simulink model "simulator_v1"  (R2025b)
settings: Solver=VariableStepAuto  StartTime=0.0  StopTime=10.0  RelTol=1e-3
values from neighbouring files (symbols this model uses):
  att_ctrl = struct    [parametrosCarga4x.m]
  payload = struct    [parametrosCarga4x.m]
  pos_ctrl = struct    [parametrosCarga4x.m]
libraries: ASK x2
settings Model: Creator=ateveraz  LastModifiedBy=ateveraz

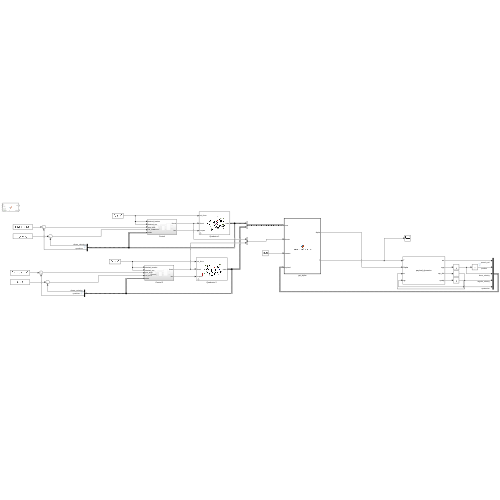
[thumbnail: Simulink's stored preview of the top-level diagram]
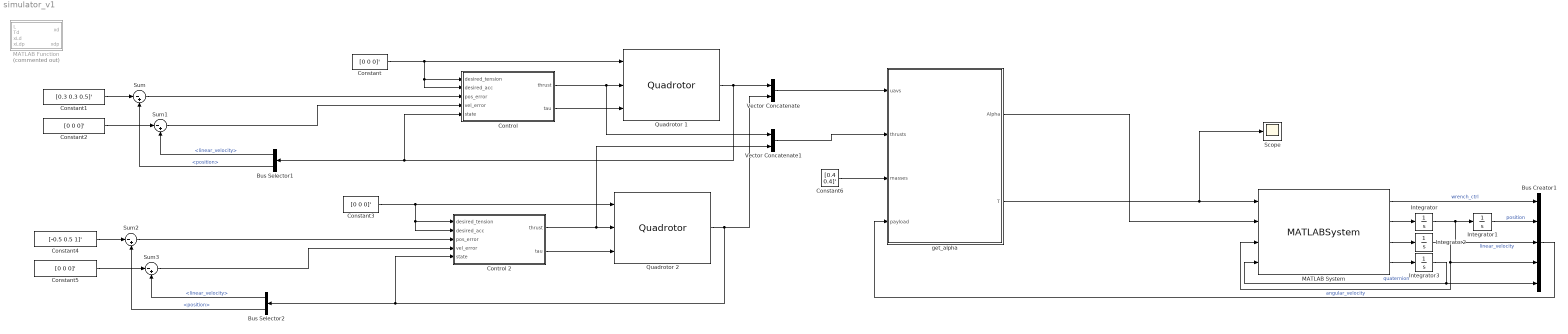
== system simulator_v1 ==
  Bus Creator1 : BusCreator  Inputs=5  OutDataTypeStr=Bus: payload_state  NonVirtualBus=on
  Bus Selector1 : BusSelector  OutputSignals=linear_velocity,position
  Bus Selector2 : BusSelector  OutputSignals=linear_velocity,position
  Constant{,2..3,5} (4 alike) : Constant  Value=[0 0 0]'
  Constant1 : Constant  Value=[0.3 0.3 0.5]'
  Constant4 : Constant  Value=[-0.5 0.5 1]'
  Constant6 : Constant  Value=[0.4 0.4]'
  Control : Subsystem
  Control 2 : Subsystem
  Integrator : Integrator  InitialCondition=payload.initial_linear_velocity
  Integrator1 : Integrator  InitialCondition=payload.initial_position
  Integrator2 : Integrator  InitialCondition=payload.initial_angular_velocity
  Integrator3 : Integrator  InitialCondition=payload.initial_quaternion
  MATLAB Function : MATLAB Function  Commented=on  TreatAsAtomicUnit=on
  MATLAB System : MATLABSystem  System=payload_dynamics  mass=payload.mass  inertia_matrix=payload.inertia_matrix  Rattach=payload.Rattach  N=payload.number_uav  SimulateUsing=Code generation
      mask Type: payload_dynamics
  Quadrotor 1 : ASK/Quadrotor  mass=uav1.mass  inertia_matrix=uav1.inertia_matrix  pos0=uav1.initial_position  vel0=uav1.initial_linear_velocity  omega0=uav1.initial_angular_velocity  quat0=uav1.initial_quaternion
      settings: SourceProductName=ASK
  Quadrotor 2 : ASK/Quadrotor  mass=uav2.mass  inertia_matrix=uav2.inertia_matrix  pos0=uav2.initial_position  vel0=uav2.initial_linear_velocity  omega0=uav2.initial_angular_velocity  quat0=uav2.initial_quaternion
      settings: SourceProductName=ASK
  Scope : Scope
      settings: ActiveDisplayYMinimum=-0.99383862161524794  ActiveDisplayYMaximum=8.9445475945372337
  Sum{,1..3} (4 alike) : Sum  Inputs=|-+
  Vector Concatenate : Concatenate
  Vector Concatenate1 : Concatenate
  get_alpha : MATLAB Function  TreatAsAtomicUnit=on
  wires:
  Bus Selector1/2 -> Sum/2  "<position>"
  Bus Selector1/1 -> Sum1/2  "<linear_velocity>"
  Quadrotor 1/1 -> Vector Concatenate/1, Control/5(state), Bus Selector1/1
  Sum/1 -> Control/3(pos_error)
  Sum1/1 -> Control/4(vel_error)
  Constant/1 -> Quadrotor 1/1, Control/1(desired_tension), Control/2(desired_acc)
  Constant1/1 -> Sum/1
  Constant2/1 -> Sum1/1
  Control/1(thrust) -> Vector Concatenate1/1, Quadrotor 1/2
  Control/2(tau) -> Quadrotor 1/3
  MATLAB System/2 -> Integrator/1
  Integrator/1 -> Integrator1/1, Bus Creator1/3  "linear_velocity"
  MATLAB System/3 -> Integrator2/1
  MATLAB System/4 -> Integrator3/1
  Integrator3/1 -> Bus Creator1/5, MATLAB System/4  "quaternion"
  Integrator2/1 -> Bus Creator1/4, MATLAB System/3  "angular_velocity"
  MATLAB System/1 -> Bus Creator1/1  "wrench_ctrl"
  Integrator1/1 -> Bus Creator1/2  "position"
  Control 2/2(tau) -> Quadrotor 2/3
  Control 2/1(thrust) -> Vector Concatenate1/2, Quadrotor 2/2
  Constant5/1 -> Sum3/1
  Constant4/1 -> Sum2/1
  Constant3/1 -> Control 2/2(desired_acc), Control 2/1(desired_tension), Quadrotor 2/1
  Sum3/1 -> Control 2/4(vel_error)
  Sum2/1 -> Control 2/3(pos_error)
  Quadrotor 2/1 -> Bus Selector2/1, Control 2/5(state), Vector Concatenate/2
  Bus Selector2/1 -> Sum3/2  "<linear_velocity>"
  Bus Selector2/2 -> Sum2/2  "<position>"
  Vector Concatenate/1 -> get_alpha/1(uavs)
  Vector Concatenate1/1 -> get_alpha/2(thrusts)
  Constant6/1 -> get_alpha/3(masses)
  get_alpha/2(T) -> Scope/1, MATLAB System/1
  get_alpha/1(Alpha) -> MATLAB System/2
  Bus Creator1/1 -> get_alpha/4(payload)

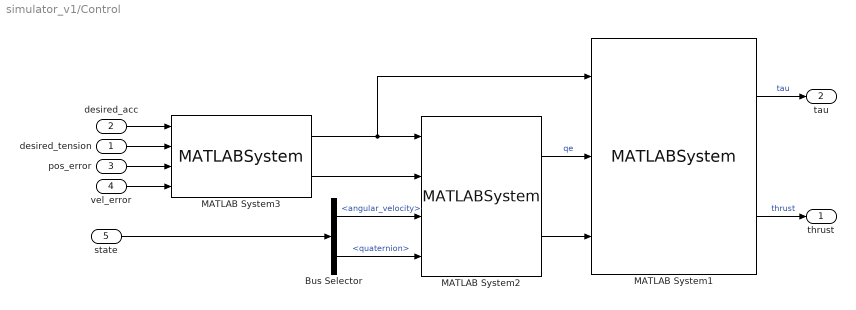
== system simulator_v1/Control ==
  desired_tension : Inport
  desired_acc : Inport  Port=2
  pos_error : Inport  Port=3
  vel_error : Inport  Port=4
  state : Inport  Port=5
  Bus Selector : BusSelector  OutputSignals=angular_velocity,quaternion
  MATLAB System1 : MATLABSystem  System=AttitudeController  Kd=att_ctrl.Kd  beta=att_ctrl.beta  gamma=att_ctrl.gamma  rho=att_ctrl.rho  SimulateUsing=Code generation
      mask Type: AttitudeController
  MATLAB System2 : MATLABSystem  System=DesiredAttitude  SimulateUsing=Code generation
      mask Type: DesiredAttitude
  MATLAB System3 : MATLABSystem  System=PositionController  Kd=pos_ctrl.Kd  alpha=pos_ctrl.alpha  mass=pos_ctrl.mass  SimulateUsing=Interpreted execution
      mask Type: PositionController
  thrust : Outport
  tau : Outport  Port=2
  wires:
  MATLAB System2/2 -> MATLAB System1/3
  MATLAB System2/1 -> MATLAB System1/2  "qe"
  Bus Selector/1 -> MATLAB System2/3  "<angular_velocity>"
  Bus Selector/2 -> MATLAB System2/4  "<quaternion>"
  MATLAB System3/2 -> MATLAB System2/2
  state/1 -> Bus Selector/1
  MATLAB System3/1 -> MATLAB System1/1, MATLAB System2/1
  pos_error/1 -> MATLAB System3/3
  vel_error/1 -> MATLAB System3/4
  desired_tension/1 -> MATLAB System3/2
  desired_acc/1 -> MATLAB System3/1
  MATLAB System1/1 -> tau/1  "tau"
  MATLAB System1/2 -> thrust/1  "thrust"

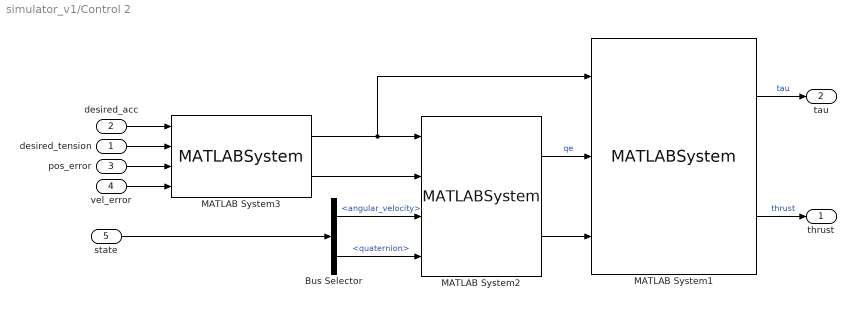
== system simulator_v1/Control 2 ==
  desired_tension : Inport
  desired_acc : Inport  Port=2
  pos_error : Inport  Port=3
  vel_error : Inport  Port=4
  state : Inport  Port=5
  Bus Selector : BusSelector  OutputSignals=angular_velocity,quaternion
  MATLAB System1 : MATLABSystem  System=AttitudeController  Kd=att_ctrl.Kd  beta=att_ctrl.beta  gamma=att_ctrl.gamma  rho=att_ctrl.rho  SimulateUsing=Code generation
      mask Type: AttitudeController
  MATLAB System2 : MATLABSystem  System=DesiredAttitude  SimulateUsing=Code generation
      mask Type: DesiredAttitude
  MATLAB System3 : MATLABSystem  System=PositionController  Kd=pos_ctrl.Kd  alpha=pos_ctrl.alpha  mass=pos_ctrl.mass  SimulateUsing=Interpreted execution
      mask Type: PositionController
  thrust : Outport
  tau : Outport  Port=2
  wires:
  MATLAB System1/2 -> thrust/1  "thrust"
  MATLAB System1/1 -> tau/1  "tau"
  desired_acc/1 -> MATLAB System3/1
  desired_tension/1 -> MATLAB System3/2
  vel_error/1 -> MATLAB System3/4
  pos_error/1 -> MATLAB System3/3
  MATLAB System3/1 -> MATLAB System2/1, MATLAB System1/1
  state/1 -> Bus Selector/1
  MATLAB System3/2 -> MATLAB System2/2
  Bus Selector/2 -> MATLAB System2/4  "<quaternion>"
  Bus Selector/1 -> MATLAB System2/3  "<angular_velocity>"
  MATLAB System2/1 -> MATLAB System1/2  "qe"
  MATLAB System2/2 -> MATLAB System1/3

== matlab function simulator_v1/get_alpha ==
  data: uavs input; thrusts input; masses input; Alpha output; payload input; T output
function [Alpha, T] = compute_cable_states(uavs, thrusts, masses, payload)
    g  = 9.81;
    e3 = [0;0;1];

    N = length(uavs);

    Alpha = zeros(3,N);
    T = zeros(N,1);

    for i = 1:N
        mi = masses(i);

        dist = payload.position - uavs(i).position;
        nd = norm(dist);

        if nd < 1e-8
            Alpha(:,i) = [0;0;1];
            T(i) = 0;
            continue;
        end

        alpha_i = dist / nd;
        Alpha(:,i) = alpha_i;

        ui = thrusts(i) * rotate_by_quat(uavs(i).quaternion, e3);

        Ti = alpha_i.' * (mi * uavs(i).linear_acceleration + ui - mi * g * e3);

        if Ti < 0
            Ti = 0;
        end

        T(i) = Ti;
    end
end

%% ===== Helpers =====
function vI = rotate_by_quat(q, v)
    vq = [0; v(:)];
    tmp = quat_mult(q, vq);
    tmp = quat_mult(tmp, quat_conj(q));
    vI = tmp(2:4);
end

function q = quat_conj(qin)
    q = [qin(1); -qin(2:4)];
end

function q = quat_mult(p, r)
    q = [ p(1)*r(1) - p(2:4).'*r(2:4);
          p(1)*r(2:4) + r(1)*p(2:4) + cross(p(2:4), r(2:4)) ];
end

== matlab function simulator_v1/MATLAB Function ==
  data: L input; xd output; Td input; xLd input; xLdp input; xdp output
function [xd, xdp] = fcn(L,  Td, xLd, xLdp)
    alpha = zeros(3,1);
    if (norm(Td)~=0)
        alpha = Td/norm(Td);
    end
    xd = xLd - L*alpha;
    xdp = xLdp;
end
